simulink model "k1visetmxmon"  (Simulink 8.8)
settings: Solver=VariableStepAuto  StartTime=0.0  StopTime=10.0  RelTol=1e-3  EnableMultiTasking=on
libraries: cdsAdcx0 x1, cdsAdcx1 x1, cdsAdcx2 x1, VISMON_MASTER x1, cdsIPCx x1, cdsModelRate x1, cdsParameters x1
settings Model: SuppressorTable=22 serialization::archive 11 0 3 0 0 0 11 0  Creator=controls  LastModifiedBy=controls
settings DataIOCC: SaveFormat=Dataset  SignalLoggingSaveFormat=Dataset
settings DebuggingCC: UnderspecifiedInitializationDetection=Simplified  MergeDetectMultiDrivingBlocksExec=error  FcnCallInpInsideContextMsg=error  AllowSymbolicDim=off  StateNameClashWarn=none
settings HardwareCC: ProdBitPerPointer=64  ProdBitPerSizeT=64  ProdBitPerPtrDiffT=64  ProdLargestAtomicFloat=Float  ProdIntDivRoundTo=Zero  ProdEndianess=LittleEndian  ProdWordSize=64  ProdHWDeviceType=Intel->x86-64 (Windows64)
settings GRTTargetCC: GeneratePreprocessorConditionals=Use local settings  CombineOutputUpdateFcns=on  GRTInterface=off

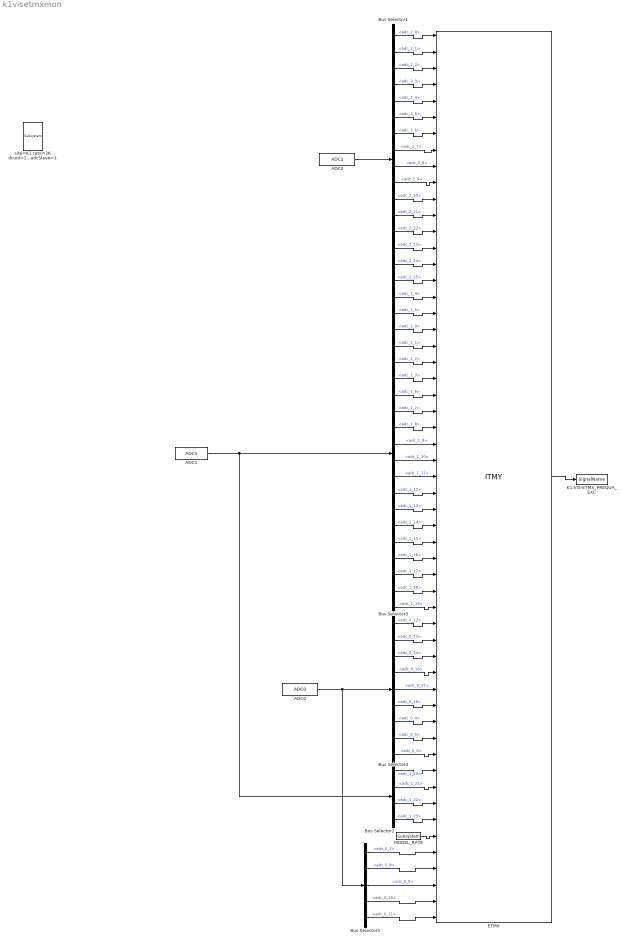
== system k1visetmxmon ==
  ADC0 : cdsAdcx0/ADC0  Tag=cdsAdc  Description=|
      | type-GSC_16AI64SSA
      | card_num=0
      settings: AttributesFormatString=%<Description>\n%<Tag>
  ADC1 : cdsAdcx1/ADC1  Tag=cdsAdc  Description=|
      | type-GSC_16AI64SSA
      | card_num=1
      settings: AttributesFormatString=%<Description>\n%<Tag>
  ADC2 : cdsAdcx2/ADC2  Tag=cdsAdc  Description=|
      | type-GSC_16AI64SSA
      | card_num=2
      settings: AttributesFormatString=%<Description>\n%<Tag>
  Bus Selector1 : BusSelector  Description=ADC Selector  OutputSignals=adc_2_0,adc_2_1,adc_2_2,adc_2_3,adc_2_4,adc_2_5,adc_2_6,adc_2_7,adc_2_8,adc_2_9,adc_2_10,adc_2_11,adc_2_12,adc_2_13,adc_2_14,adc_2_15
      settings: AttributesFormatString=%<Description>
  Bus Selector2 : BusSelector  OutputSignals=adc_1_20,adc_1_21,adc_1_22,adc_1_23
  Bus Selector3 : BusSelector  OutputSignals=adc_1_4,adc_1_5,adc_1_0,adc_1_1,adc_1_2,adc_1_3,adc_1_6,adc_1_7,adc_1_8,adc_1_9,adc_1_10,adc_1_11,adc_1_12,adc_1_13,adc_1_14,adc_1_15,adc_1_16,adc_1_17,adc_1_18,adc_1_19
  Bus Selector4 : BusSelector  OutputSignals=adc_0_12,adc_0_13,adc_0_14,adc_0_16,adc_0_17,adc_0_18,adc_0_4,adc_0_5,adc_0_6
  Bus Selector5 : BusSelector  OutputSignals=adc_0_7,adc_0_8,adc_0_9,adc_0_10,adc_0_11
  ETMX : VISMON_MASTER/ITMY
  K1:VIS-ETMX_PREQUA_EXC : cdsIPCx/SignalName  Tag=cdsIPCx_SHMEM  Description=Inter-Process Communication via Shared memory.
      settings: AttributesFormatString=%<Tag>
  MODEL_RATE : cdsModelRate/Subsystem  Tag=cdsModelRate
      settings: AttributesFormatString=%<Tag>
  site=K1 rate=2K dcuid=104 host=k1ex1 specific_cpu=4 adcSlave=1 : cdsParameters/Subsystem  Tag=cdsParameters  Description=|
      | Purpose:                                                                                                                                                                                                                                
      | Provide system parameters to the FE code generator to properly configure the generated EPICS names, rep rate of the FE controller, and the Data Acquisition node ID for proper storage of data from this FE controller.                 
      |                                                                                                                                                                                                                                         
      | Useage:                                                                                                                                                                                                                                 
      | The part NAME field is used to identify the FE parameters. It must be of the form:                                                                                                                                                      
      | site=                                                                                                                                                                                                                                   
      | rate=                                                                                                                                                                                                                                   
      | dcuid=                                                                                                                                                                                                                                  
      |                                                                                                                                                                                                                                         
      | Where:                                                                                                                                                                                                                                  
      | site= argument may be H1, H2, L1, M1, G1, either as a single argument or multiple, for example site=H1,H2. These are the only names allowed. These will become the first two characters of all EPICS and signal names (for example G1:).
      |                                                                                                                                                                                                                                         
      | rate= may be 2K, 16K, 32K, or 64K                                                                                                                                                                                                       
      |                                                                                                                                                                                                                                         
      | dcuid= is site specific ie it must be unique at each site.
      settings: AttributesFormatString=%<Tag>
  wires:
  ADC2/1 -> Bus Selector1/1
  Bus Selector1/1 -> ETMX/1  "<adc_2_0>"
  Bus Selector1/2 -> ETMX/2  "<adc_2_1>"
  Bus Selector1/3 -> ETMX/3  "<adc_2_2>"
  Bus Selector1/4 -> ETMX/4  "<adc_2_3>"
  Bus Selector1/5 -> ETMX/5  "<adc_2_4>"
  Bus Selector1/6 -> ETMX/6  "<adc_2_5>"
  Bus Selector1/7 -> ETMX/7  "<adc_2_6>"
  Bus Selector1/8 -> ETMX/8  "<adc_2_7>"
  Bus Selector1/9 -> ETMX/9  "<adc_2_8>"
  Bus Selector1/10 -> ETMX/10  "<adc_2_9>"
  Bus Selector1/11 -> ETMX/11  "<adc_2_10>"
  Bus Selector1/12 -> ETMX/12  "<adc_2_11>"
  Bus Selector1/13 -> ETMX/13  "<adc_2_12>"
  Bus Selector1/14 -> ETMX/14  "<adc_2_13>"
  Bus Selector1/15 -> ETMX/15  "<adc_2_14>"
  Bus Selector1/16 -> ETMX/16  "<adc_2_15>"
  MODEL_RATE/1 -> ETMX/50
  ETMX/1 -> K1:VIS-ETMX_PREQUA_EXC/1
  ADC1/1 -> Bus Selector2/1, Bus Selector3/1
  Bus Selector3/1 -> ETMX/17  "<adc_1_4>"
  Bus Selector3/2 -> ETMX/18  "<adc_1_5>"
  Bus Selector3/3 -> ETMX/19  "<adc_1_0>"
  Bus Selector3/4 -> ETMX/20  "<adc_1_1>"
  Bus Selector3/5 -> ETMX/21  "<adc_1_2>"
  Bus Selector3/6 -> ETMX/22  "<adc_1_3>"
  Bus Selector3/7 -> ETMX/23  "<adc_1_6>"
  Bus Selector3/8 -> ETMX/24  "<adc_1_7>"
  Bus Selector3/9 -> ETMX/25  "<adc_1_8>"
  Bus Selector3/10 -> ETMX/26  "<adc_1_9>"
  Bus Selector3/11 -> ETMX/27  "<adc_1_10>"
  Bus Selector3/12 -> ETMX/28  "<adc_1_11>"
  Bus Selector3/13 -> ETMX/29  "<adc_1_12>"
  Bus Selector3/14 -> ETMX/30  "<adc_1_13>"
  Bus Selector3/15 -> ETMX/31  "<adc_1_14>"
  Bus Selector3/16 -> ETMX/32  "<adc_1_15>"
  Bus Selector3/17 -> ETMX/33  "<adc_1_16>"
  Bus Selector3/18 -> ETMX/34  "<adc_1_17>"
  Bus Selector3/19 -> ETMX/35  "<adc_1_18>"
  Bus Selector3/20 -> ETMX/36  "<adc_1_19>"
  ADC0/1 -> Bus Selector5/1, Bus Selector4/1
  Bus Selector4/1 -> ETMX/37  "<adc_0_12>"
  Bus Selector4/2 -> ETMX/38  "<adc_0_13>"
  Bus Selector4/3 -> ETMX/39  "<adc_0_14>"
  Bus Selector4/4 -> ETMX/40  "<adc_0_16>"
  Bus Selector4/5 -> ETMX/41  "<adc_0_17>"
  Bus Selector4/6 -> ETMX/42  "<adc_0_18>"
  Bus Selector4/7 -> ETMX/43  "<adc_0_4>"
  Bus Selector4/8 -> ETMX/44  "<adc_0_5>"
  Bus Selector4/9 -> ETMX/45  "<adc_0_6>"
  Bus Selector2/1 -> ETMX/46  "<adc_1_20>"
  Bus Selector2/2 -> ETMX/47  "<adc_1_21>"
  Bus Selector2/3 -> ETMX/48  "<adc_1_22>"
  Bus Selector2/4 -> ETMX/49  "<adc_1_23>"
  Bus Selector5/2 -> ETMX/52  "<adc_0_8>"
  Bus Selector5/3 -> ETMX/53  "<adc_0_9>"
  Bus Selector5/4 -> ETMX/54  "<adc_0_10>"
  Bus Selector5/5 -> ETMX/55  "<adc_0_11>"
  Bus Selector5/1 -> ETMX/51  "<adc_0_7>"
